simulink model "zad2"  (Simulink 7.5)
settings: Solver=ode45  StartTime=0.0  StopTime=30000  RelTol=1e-3
settings Model: Creator=Maja  LastModifiedBy=Marin
settings DebuggingCC: FcnCallInpInsideContextMsg=Enable All
settings GRTTargetCC: CombineOutputUpdateFcns=on

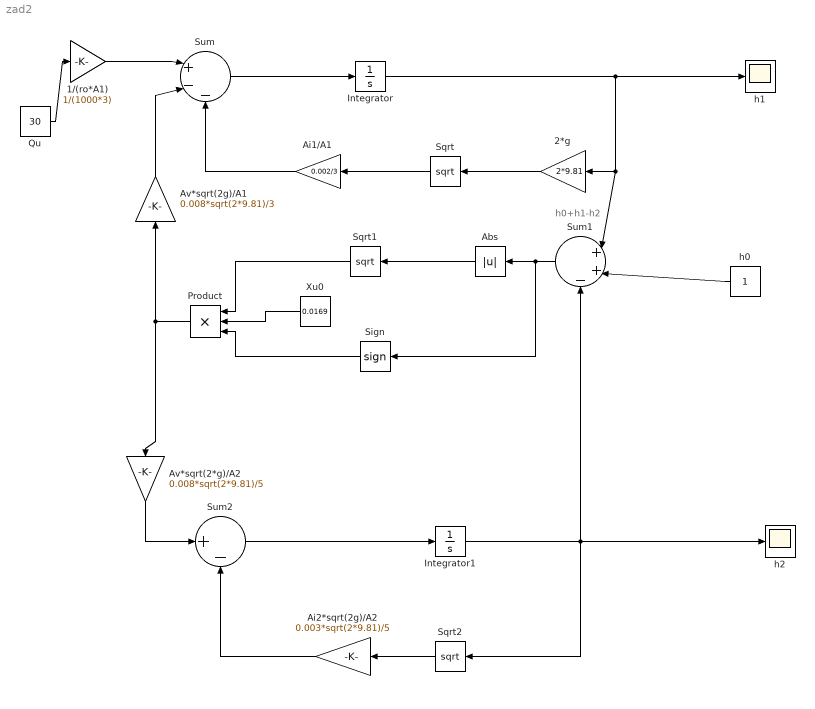
== system zad2 ==
  note: h0+h1-h2
  1/(ro*A1) : Gain  Gain=1/(1000*3)
  2*g : Gain  Gain=2*9.81
  Abs : Abs
  Ai1/A1 : Gain  Gain=0.002/3
  Ai2*sqrt(2g)/A2 : Gain  Gain=0.003*sqrt(2*9.81)/5
  Av*sqrt(2*g)/A2 : Gain  Gain=0.008*sqrt(2*9.81)/5
  Av*sqrt(2g)/A1 : Gain  Gain=0.008*sqrt(2*9.81)/3
  Integrator : Integrator
  Integrator1 : Integrator
  Product : Product  Inputs=3  RndMeth=Zero
  Qu : Constant  Value=30
  Sign : Signum
  Sqrt : Sqrt  AlgorithmType=Exact  SaturateOnIntegerOverflow=on
  Sqrt1 : Sqrt  AlgorithmType=Exact  SaturateOnIntegerOverflow=on
  Sqrt2 : Sqrt  AlgorithmType=Exact  SaturateOnIntegerOverflow=on
  Sum : Sum  Inputs=|+--
  Sum1 : Sum  Inputs=|++-
  Sum2 : Sum  Inputs=|+-
  Xu0 : Constant  Value=0.0169
  h0 : Constant
  h1 : Scope
  h2 : Scope
  wires:
  1/(ro*A1)/1 -> Sum/1
  Sum/1 -> Integrator/1
  Integrator/1 -> 2*g/1, Sum1/1, h1/1
  Ai1/A1/1 -> Sum/3
  h0/1 -> Sum1/2
  Sum1/1 -> Abs/1, Sign/1
  Product/1 -> Av*sqrt(2g)/A1/1, Av*sqrt(2*g)/A2/1
  Sum2/1 -> Integrator1/1
  Integrator1/1 -> h2/1, Sum1/3, Sqrt2/1
  Ai2*sqrt(2g)/A2/1 -> Sum2/2
  Qu/1 -> 1/(ro*A1)/1
  Sqrt2/1 -> Ai2*sqrt(2g)/A2/1
  Abs/1 -> Sqrt1/1
  Sqrt/1 -> Ai1/A1/1
  2*g/1 -> Sqrt/1
  Av*sqrt(2*g)/A2/1 -> Sum2/1
  Av*sqrt(2g)/A1/1 -> Sum/2
  Sign/1 -> Product/3
  Sqrt1/1 -> Product/1
  Xu0/1 -> Product/2
